simulink model "Basic_Switch"  (R2018b)
settings: Solver=VariableStepAuto  StartTime=0.0  StopTime=10.0  RelTol=1e-3
undefined symbols (not defined in the file): a
libraries: simulink x2
settings Model: Creator=nswat  LastModifiedBy=nswat

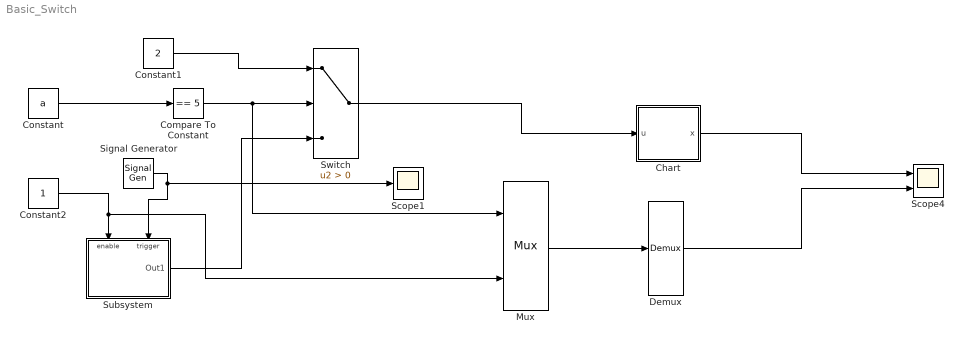
== system Basic_Switch ==
  Chart : Stateflow chart  TreatAsAtomicUnit=on
  Compare To Constant : simulink/Logic and Bit Operations/Compare To Constant  relop===  const=5  OutDataTypeStr=boolean
  Constant : Constant  Value=a
  Constant1 : Constant  Value=2
  Constant2 : Constant  OutDataTypeStr=boolean
  Demux : Demux  Outputs=1
  Mux : Mux  Inputs=2
      settings: DisplayOption=signals
  Scope1 : Scope
  Scope4 : Scope  NumInputPorts=2
  Signal Generator : SignalGenerator  WaveForm=square
  Subsystem : Subsystem
  Switch : Switch  Criteria=u2 > Threshold
  wires:
  Constant/1 -> Compare To Constant/1
  Compare To Constant/1 -> Mux/1, Switch/2
  Constant1/1 -> Switch/1
  Switch/1 -> Chart/1(u)
  Subsystem/1(Out1) -> Switch/3
  Constant2/1 -> Mux/2, Subsystem/Enable
  Signal Generator/1 -> Subsystem/Trigger, Scope1/1
  Mux/1 -> Demux/1
  Chart/1(x) -> Scope4/1
  Demux/1 -> Scope4/2

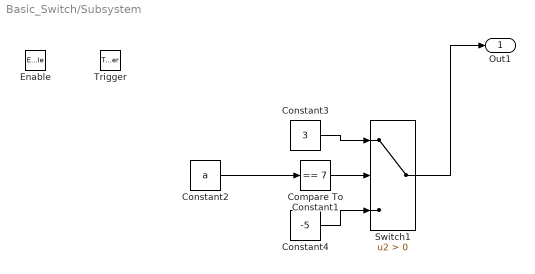
== system Basic_Switch/Subsystem ==
  Enable : EnablePort
  Trigger : TriggerPort  TriggerType=falling  VariantControl=Variant  PortDimensions=1
  Compare To Constant1 : simulink/Logic and Bit Operations/Compare To Constant  relop===  const=7  OutDataTypeStr=boolean
  Constant2 : Constant  Value=a
  Constant3 : Constant  Value=3
  Constant4 : Constant  Value=-5
  Switch1 : Switch  Criteria=u2 > Threshold
  Out1 : Outport
  wires:
  Constant3/1 -> Switch1/1
  Constant2/1 -> Compare To Constant1/1
  Compare To Constant1/1 -> Switch1/2
  Constant4/1 -> Switch1/3
  Switch1/1 -> Out1/1

== stateflow chart Basic_Switch/Chart ==
  (default) -> (junction 19) [order 2] : [u<0]
  (default) -> (junction 14) [order 1] : [u>0]
  (junction 19) -> (junction 21) : {x=-u}
  (junction 14) -> (junction 18) : {x=u}
  data: u input; x output
